simulink subsystem "CurrentForMotor"  (R2019b)
settings: Solver=VariableStepAuto  StartTime=0.0  StopTime=10.0  RelTol=1e-3
values from neighbouring files (symbols this model uses):
  k = 0.035    [part1.m]
settings Model: Creator=ovi  LastModifiedBy=ovi

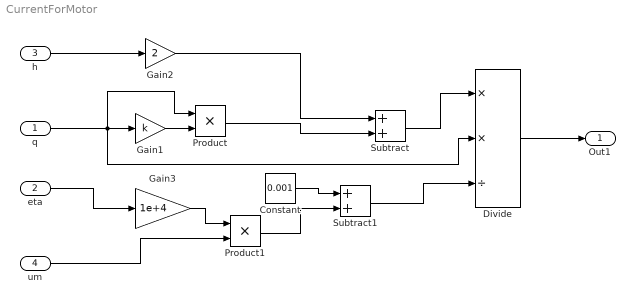
== system CurrentForMotor ==
  q : Inport
  eta : Inport  Port=2
  "h " : Inport  Port=3
  um : Inport  Port=4
  Constant : Constant  Value=0.001
  Divide : Product  Inputs=**/
  Gain1 : Gain  Gain=k
  Gain2 : Gain  Gain=2
  Gain3 : Gain  Gain=1e+4
  Product : Product
  Product1 : Product
  Subtract : Sum
  Subtract1 : Sum
  Out1 : Outport
  wires:
  "h "/1 -> Gain2/1
  q/1 -> Divide/2, Product/1, Gain1/1
  Gain1/1 -> Product/2
  Gain3/1 -> Product1/1
  eta/1 -> Gain3/1
  um/1 -> Product1/2
  Product1/1 -> Subtract1/2
  Product/1 -> Subtract/2
  Gain2/1 -> Subtract/1
  Subtract1/1 -> Divide/3
  Subtract/1 -> Divide/1
  Constant/1 -> Subtract1/1
  Divide/1 -> Out1/1
